simulink model "MCS_STD_FSBB_MODEL_2022b"  (R2022b)
settings: Solver=VariableStepAuto  StartTime=0.0  StopTime=2  RelTol=1e-3
PostLoadFcn:
  | gmp_model_file=get_param(bdroot,'FileName'); if isempty(gmp_model_file), error('GMP:SDPE:ModelPath','The model must be saved before SDPE initialization.'); end; gmp_model_dir=fileparts(gmp_model_file); run(fullfile(gmp_model_dir,'sdpe_mgr','ctrl_settings_matlab_init.m')); gmp_matlab_release=matlabRelease; gmp_repo_root=fullfile(gmp_model_dir,'..','..','..','..','..'); addpath(fullfile(gmp_repo_root,'slib','install_path',gmp_matlab_release.Release,'src')); clear gmp_model_file gmp_model_dir gmp_matlab_release gmp_repo_root;
InitFcn:
  | gmp_model_file=get_param(bdroot,'FileName'); if isempty(gmp_model_file), error('GMP:SDPE:ModelPath','The model must be saved before SDPE initialization.'); end; gmp_model_dir=fileparts(gmp_model_file); run(fullfile(gmp_model_dir,'sdpe_mgr','ctrl_settings_matlab_init.m')); gmp_matlab_release=matlabRelease; gmp_repo_root=fullfile(gmp_model_dir,'..','..','..','..','..'); addpath(fullfile(gmp_repo_root,'slib','install_path',gmp_matlab_release.Release,'src')); clear gmp_model_file gmp_model_dir gmp_matlab_release gmp_repo_root;
undefined symbols (not defined in the file or in its folder): CTRL_ADC_RESOLUTION, CTRL_ADC_VOLTAGE_REF, CTRL_FSBB_IIN_BIAS, CTRL_FSBB_IIN_SENSITIVITY, CTRL_FSBB_IL_BIAS, CTRL_FSBB_IL_SENSITIVITY, CTRL_FSBB_IOUT_BIAS, CTRL_FSBB_IOUT_SENSITIVITY, CTRL_FSBB_VIN_BIAS, CTRL_FSBB_VIN_SENSITIVITY, CTRL_FSBB_VOUT_BIAS, CTRL_FSBB_VOUT_SENSITIVITY, CTRL_PWM_CMP_MAX, CTRL_PWM_DEADBAND_CMP, FSBB_INPUT_VOLTAGE_NOMINAL, FSBB_MODEL_DIODE_RON, FSBB_MODEL_DIODE_VF, FSBB_MODEL_MOSFET_RON, FSBB_MODEL_SNUBBER_C, FSBB_MODEL_SNUBBER_R, FSBB_MODEL_SWITCH_LON, FSBB_PARAM_CIN, FSBB_PARAM_CIN_ESR, FSBB_PARAM_COUT, FSBB_PARAM_COUT_ESR, FSBB_PARAM_L, FSBB_PARAM_L_ESR, FSBB_PARAM_RLOAD_MIN, PWM_FREQ
libraries: gmp_peripheral_utilities x4, spsSeriesRLCBranchLib x4, gmp_std_model_pck x3, spsControlledVoltageSourceLib x1, gmp_sil_core_pack x1, spsGroundLib x1, spspowerguiLib x1
settings Model: SimulationMode=accelerator  Creator=javnson  LastModifiedBy=javnson
settings OptimizationCC: ReuseModelBlockBuffer=on
settings RTWCC: GPUComputeCapability=5.0

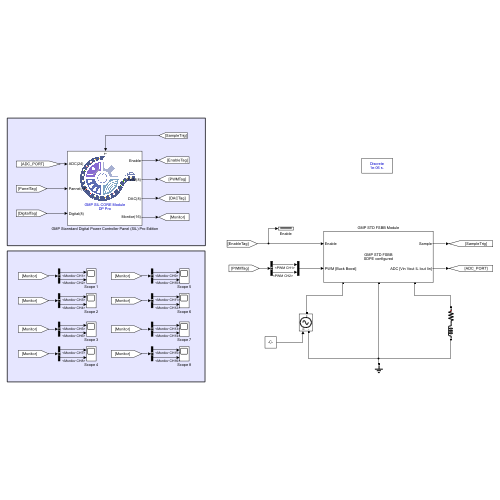
[thumbnail: Simulink's stored preview of the top-level diagram]
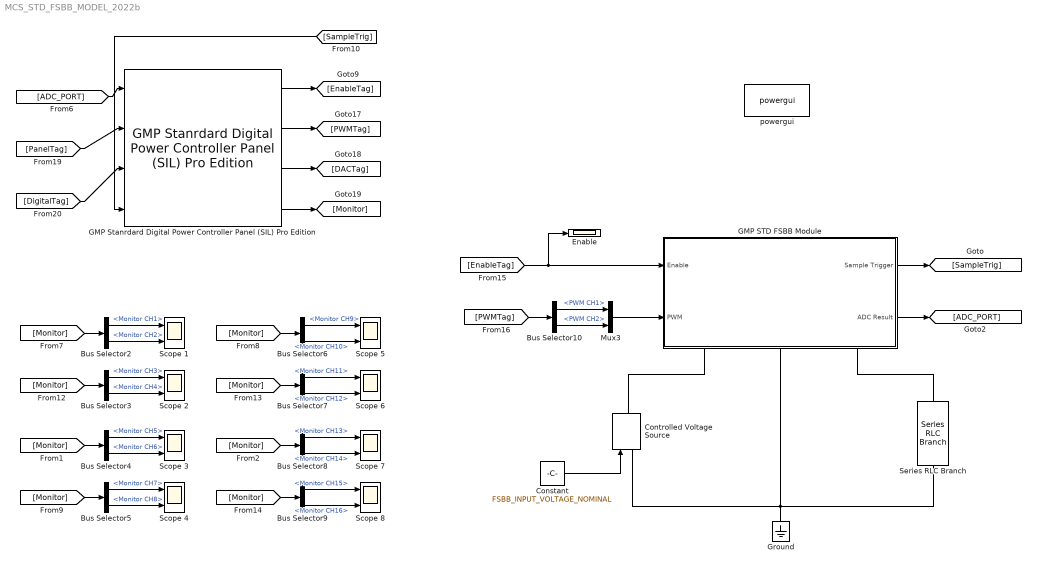
== system MCS_STD_FSBB_MODEL_2022b ==
  Bus Selector10 : BusSelector  OutputSignals=PWM CH1,PWM CH2
  Bus Selector2 : BusSelector  OutputSignals=Monitor CH1,Monitor CH2
  Bus Selector3 : BusSelector  OutputSignals=Monitor CH3,Monitor CH4
  Bus Selector4 : BusSelector  OutputSignals=Monitor CH5,Monitor CH6
  Bus Selector5 : BusSelector  OutputSignals=Monitor CH7,Monitor CH8
  Bus Selector6 : BusSelector  OutputSignals=Monitor CH9,Monitor CH10
  Bus Selector7 : BusSelector  OutputSignals=Monitor CH11,Monitor CH12
  Bus Selector8 : BusSelector  OutputSignals=Monitor CH13,Monitor CH14
  Bus Selector9 : BusSelector  OutputSignals=Monitor CH15,Monitor CH16
  Constant : Constant  Value=FSBB_INPUT_VOLTAGE_NOMINAL
  Controlled Voltage Source : spsControlledVoltageSourceLib/Controlled Voltage Source  Initialize=on  Source_Type=AC  Amplitude=0  Phase=0  Frequency=0  Measurements=None
  Enable : Scope
  GMP STD FSBB Module : Subsystem  mask{Switching_Frequency=PWM_FREQ, PWM_Compare_Max=CTRL_PWM_CMP_MAX, Deadband_Compare=CTRL_PWM_DEADBAND_CMP, Phase_Shift=0, Main_Inductance=FSBB_PARAM_L, Inductor_ESR=FSBB_PARAM_L_ESR, Input_Capacitance=FSBB_PARAM_CIN, Input_Capacitor_ESR=FSBB_PARAM_CIN_ESR, Output_Capacitance=FSBB_PARAM_COUT, Output_Capacitor_ESR=FSBB_PARAM_COUT_ESR, MOSFET_Ron=FSBB_MODEL_MOSFET_RON, Switch_Lon=FSBB_MODEL_SWITCH_LON, Diode_Ron=FSBB_MODEL_DIODE_RON, Diode_Vf=FSBB_MODEL_DIODE_VF, Snubber_R=FSBB_MODEL_SNUBBER_R, Snubber_C=FSBB_MODEL_SNUBBER_C, ADC_Bits=CTRL_ADC_RESOLUTION, ADC_Reference=CTRL_ADC_VOLTAGE_REF, ADC_Initial_Value=0, Vin_Sensor_Gain=CTRL_FSBB_VIN_SENSITIVITY, Vin_Sensor_Bias=CTRL_FSBB_VIN_BIAS, Vout_Sensor_Gain=CTRL_FSBB_VOUT_SENSITIVITY, Vout_Sensor_Bias=CTRL_FSBB_VOUT_BIAS, IL_Sensor_Gain=CTRL_FSBB_IL_SENSITIVITY, IL_Sensor_Bias=CTRL_FSBB_IL_BIAS, Iout_Sensor_Gain=CTRL_FSBB_IOUT_SENSITIVITY, Iout_Sensor_Bias=CTRL_FSBB_IOUT_BIAS, Iin_Sensor_Gain=CTRL_FSBB_IIN_SENSITIVITY, Iin_Sensor_Bias=CTRL_FSBB_IIN_BIAS}
      mask prompts: Switching_Frequency "Switching frequency (Hz)"; PWM_Compare_Max "PWM compare maximum"; Deadband_Compare "Deadband (compare counts)"; Phase_Shift "Phase shift (deg)"; Main_Inductance "Main inductance (H)"; Inductor_ESR "Inductor ESR (Ohm)"; Input_Capacitance "Input capacitance (F)"; Input_Capacitor_ESR "Input capacitor ESR (Ohm)"; Output_Capacitance "Output capacitance (F)"; Output_Capacitor_ESR "Output capacitor ESR (Ohm)"; MOSFET_Ron "MOSFET on resistance (Ohm)"; Switch_Lon "Switch series inductance (H)"; Diode_Ron "Body-diode on resistance (Ohm)"; Diode_Vf "Body-diode forward voltage (V)"; Snubber_R "Snubber resistance (Ohm)"; Snubber_C "Snubber capacitance (F)"; ADC_Bits "ADC resolution (bits)"; ADC_Reference "ADC reference (V)"; ADC_Initial_Value "Sample-and-hold initial value"; Vin_Sensor_Gain "Input-voltage sensitivity (V/V)"; Vin_Sensor_Bias "Input-voltage bias (V)"; Vout_Sensor_Gain "Output-voltage sensitivity (V/V)"; Vout_Sensor_Bias "Output-voltage bias (V)"; IL_Sensor_Gain "Inductor-current sensitivity (V/A)"; IL_Sensor_Bias "Inductor-current bias (V)"; Iout_Sensor_Gain "Boost-side/output-current sensitivity (V/A)"; Iout_Sensor_Bias "Boost-side/output-current bias (V)"; Iin_Sensor_Gain "Buck-side/input-current sensitivity (V/A)"; Iin_Sensor_Bias "Buck-side/input-current bias (V)"
      mask help: SDPE-configured four-switch buck-boost plant. ADC output order: Vin, Vout, IL, Iout (Boost side), Iin (Buck side).
      settings: PortSchema="{\"entries\":[{\"content\":{\"sides\":[{\"content\":{\"connectorIds\":[\"In1\",\"In2\"]},\"type\":\"ConnectorPlacement.EquallySpacedRectSide\",\"uuid\":\"d5d2152c-95da-402f-99b0-c218dbe2e5b0\"},{\"content\":{\"connectorIds\":[\"Out1\",\"Out2\"],\"side\":\"RIGHT\"},\"type\":\"ConnectorPlacement.EquallySpacedRectSide\",\"uuid\":\"d6dcb103-1a45-4ef6-9907-93a1989d933d\"},{\"content\":{\"side\":\"TOP\"},\"type\":\"ConnectorPlacement.EquallySpacedRectSide\",\"uuid\":\"e6268914-9f06-47c0-ace2-6fbd0fa30956\"},{\"content\":{\"connectorIds\":[\"RConn1\",\"RConn2\",\"RConn3\"],\"side\":\"BOTTOM\"},\"type\":\"ConnectorPlacement.EquallySpacedRectSide\",\"uuid\":\"d75aaae5-4ace-4756-8126-8df6a2fa5cb9\"}]},\"type\":\"ConnectorPlacement.EquallySpacedConnector\",\"uuid\":\"07c59de5-034f-4952-94ab-3f04d206adfb\"}],\"packageUris\":[\"http://schema.mathworks.com/mf0/Connector/R2020b\"],\"version\":\"1.0\"}"
      mask DialogControl PWMConfiguration_Group Prompt: PWM Configuration
      mask DialogControl PowerStage_Group Prompt: Power Stage
      mask DialogControl SemiconductorModel_Group Prompt: Semiconductor Model
      mask DialogControl ADCConfiguration_Group Prompt: ADC Configuration
      mask DialogControl VoltageSensors_Group Prompt: Voltage Sensors
      mask DialogControl CurrentSensors_Group Prompt: Current Sensors
      mask Display:
      | disp('GMP STD FSBB\nSDPE configured');
      | port_label('input',1,'Enable'); port_label('input',2,'PWM [Buck Boost]');
      | port_label('output',1,'Sample'); port_label('output',2,'ADC [Vin Vout IL Iout Iin]');
  GMP Stanrdard Digital Power Controller Panel (SIL) Pro Edition : gmp_sil_core_pack/GMP Stanrdard Digital Power Controller Panel (SIL) Pro Edition
      settings: SourceProductName=GMP SIL Core Utilities
  Ground : spsGroundLib/Ground  LConnTagsString=a
  Mux3 : Mux  Inputs=2
  Scope {1..8} (8 alike) : Scope  NumInputPorts=2
  Series RLC Branch : spsSeriesRLCBranchLib/Series RLC Branch  LConnTagsString=__new0  RConnTagsString=__new0  BranchType=RL  Resistance=FSBB_PARAM_RLOAD_MIN  Inductance=10E-6  SetiL0=off  InitialCurrent=0  Capacitance=1e-6  Setx0=off  InitialVoltage=0  Measurements=None
  powergui : spspowerguiLib/powergui  Priority=1  SimulationMode=Discrete  SampleTime=1e-6  frequency=60  Iterations=50  frequencyindice=0  Pbase=100e6  ErrMax=1e-4  UnitsV=kV  UnitsW=MW  buscounter=0  FunctionMessages=off  echomessages=off  EnableUseOfTLC=off  CurrentSourceSwitches=off  DisableSnubberDevices=off  DisableRonSwitches=off  DisableVfSwitches=off  DisplayEquations=off  AutomaticDiscreteSolvers=off  SolverType=Tustin/Backward Euler (TBE)  Interpol=off  ExternalGateDelay=off  methode=off  Ts=100  x0status=blocks  SPID=on  SwTol=0  HookPort=off  NonlinearTolerance=1e-4  nMaxIteration=100  ContinueOnMaxIteration=off  RestoreLinks=warning  ResistiveCurrentMeasurement=off  Frange=[0:2:500]  Ylog=off  Xlog=on  ShowGrid=off  save=off  variable=ZData  structure=0  ZoomFFT=off  StartTime=0.0  cycles=1  DisplayStyle=1  fundamental=60  FreqAxis=off  MaxFrequency=1000  frequencyindicesteady=1  RmsSteady=1  display=off
  wires:
  [PanelTag] -> GMP Stanrdard Digital Power Controller Panel (SIL) Pro Edition/2
  [SampleTrig] -> GMP Stanrdard Digital Power Controller Panel (SIL) Pro Edition/4
  GMP Stanrdard Digital Power Controller Panel (SIL) Pro Edition/2 -> [PWMTag]
  [ADC_PORT] -> GMP Stanrdard Digital Power Controller Panel (SIL) Pro Edition/1
  GMP Stanrdard Digital Power Controller Panel (SIL) Pro Edition/4 -> [Monitor]
  GMP Stanrdard Digital Power Controller Panel (SIL) Pro Edition/1 -> [EnableTag]
  GMP Stanrdard Digital Power Controller Panel (SIL) Pro Edition/3 -> [DACTag]
  [DigitalTag] -> GMP Stanrdard Digital Power Controller Panel (SIL) Pro Edition/3
  Bus Selector8/2 -> Scope 7/2  "<Monitor CH14>"
  Bus Selector2/2 -> Scope 1/2  "<Monitor CH2>"
  Bus Selector4/2 -> Scope 3/2  "<Monitor CH6>"
  Bus Selector3/1 -> Scope 2/1  "<Monitor CH3>"
  [Monitor] -> Bus Selector4/1
  [Monitor] -> Bus Selector7/1
  Bus Selector2/1 -> Scope 1/1  "<Monitor CH1>"
  Bus Selector5/1 -> Scope 4/1  "<Monitor CH7>"
  [Monitor] -> Bus Selector3/1
  Bus Selector8/1 -> Scope 7/1  "<Monitor CH13>"
  Bus Selector3/2 -> Scope 2/2  "<Monitor CH4>"
  Bus Selector4/1 -> Scope 3/1  "<Monitor CH5>"
  Bus Selector7/1 -> Scope 6/1  "<Monitor CH11>"
  [Monitor] -> Bus Selector5/1
  [Monitor] -> Bus Selector8/1
  [Monitor] -> Bus Selector6/1
  Bus Selector6/1 -> Scope 5/1  "<Monitor CH9>"
  Bus Selector5/2 -> Scope 4/2  "<Monitor CH8>"
  [Monitor] -> Bus Selector2/1
  Bus Selector7/2 -> Scope 6/2  "<Monitor CH12>"
  Bus Selector6/2 -> Scope 5/2  "<Monitor CH10>"
  Bus Selector9/1 -> Scope 8/1  "<Monitor CH15>"
  [Monitor] -> Bus Selector9/1
  Bus Selector9/2 -> Scope 8/2  "<Monitor CH16>"
  GMP STD FSBB Module/1(Sample Trigger) -> [SampleTrig]
  GMP STD FSBB Module/2(ADC Result) -> [ADC_PORT]
  [EnableTag] -> GMP STD FSBB Module/1(Enable), Enable/1
  Bus Selector10/1 -> Mux3/1  "<PWM CH1>"
  Bus Selector10/2 -> Mux3/2  "<PWM CH2>"
  Mux3/1 -> GMP STD FSBB Module/2(PWM)
  [PWMTag] -> Bus Selector10/1
  Constant/1 -> Controlled Voltage Source/1
  connections:
  Controlled Voltage Source/RConn1 -- GMP STD FSBB Module/RConn1
  Series RLC Branch/RConn1 -- GMP STD FSBB Module/RConn2 -- Ground/LConn1 -- Controlled Voltage Source/LConn1
  Series RLC Branch/LConn1 -- GMP STD FSBB Module/RConn3

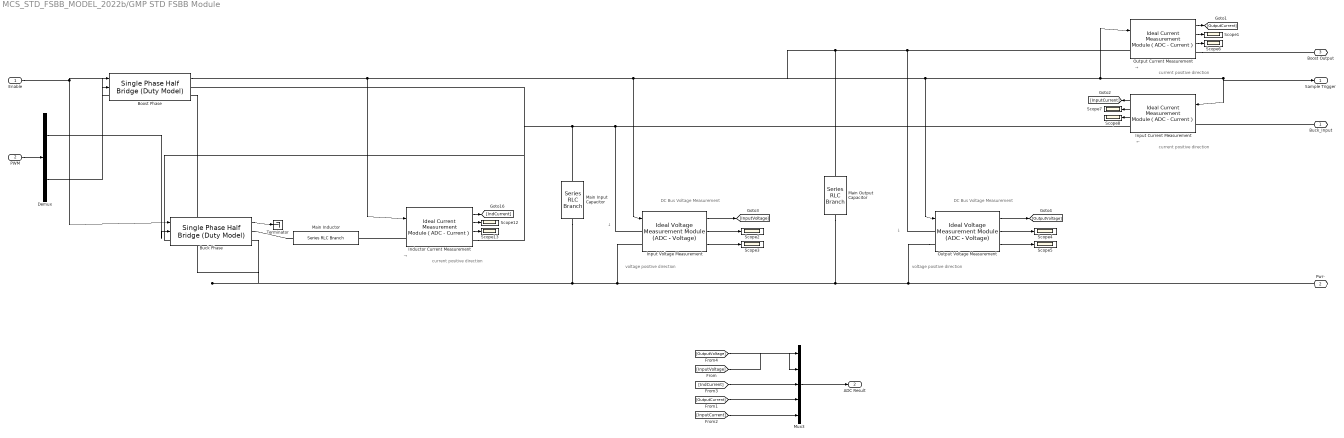
== system MCS_STD_FSBB_MODEL_2022b/GMP STD FSBB Module ==
  note: →
  note: current positive direction
  note: DC Bus Voltage Measurement
  note: ↓
  note: voltage positive direction
  note: voltage positive direction
  note: ↓
  note: DC Bus Voltage Measurement
  note: current positive direction
  note: →
  note: ←
  note: current positive direction
  Enable : Inport
  PWM : Inport  Port=2
  Boost Phase : gmp_peripheral_utilities/Single Phase Half Bridge (Duty Model)  fswitch=Switching_Frequency  CMP_MAX=PWM_Compare_Max  Deadband_Upper=Deadband_Compare  Deadband_Lower=Deadband_Compare  Deadband_us=NaN  phase_shift=Phase_Shift  R_mosfet_on=MOSFET_Ron  Lon=Switch_Lon  Rd=Diode_Ron  Vf=Diode_Vf  Rs=Snubber_R  Cs=Snubber_C
      settings: SourceProductName=Virtual Peripheral Utilities
  Buck Phase : gmp_peripheral_utilities/Single Phase Half Bridge (Duty Model)  fswitch=Switching_Frequency  CMP_MAX=PWM_Compare_Max  Deadband_Upper=Deadband_Compare  Deadband_Lower=Deadband_Compare  Deadband_us=NaN  phase_shift=Phase_Shift  R_mosfet_on=MOSFET_Ron  Lon=Switch_Lon  Rd=Diode_Ron  Vf=Diode_Vf  Rs=Snubber_R  Cs=Snubber_C
      settings: SourceProductName=Virtual Peripheral Utilities
  Demux : Demux  Outputs=2
  Inductor Current Measurement : gmp_std_model_pck/Buck (GMP STD MDL)/Ideal Current Measurement Module（ADC - Current）  ADC_GAIN=IL_Sensor_Gain  ADC_BIT=ADC_Bits  ADC_REFERENCE=ADC_Reference  ADC_BIAS=IL_Sensor_Bias  ADC_INIT=ADC_Initial_Value
      settings: SourceProductName=GMP Control Plant Utilities
  Input Current Measurement : gmp_std_model_pck/Buck (GMP STD MDL)/Ideal Current Measurement Module（ADC - Current）  ADC_GAIN=Iin_Sensor_Gain  ADC_BIT=ADC_Bits  ADC_REFERENCE=ADC_Reference  ADC_BIAS=Iin_Sensor_Bias  ADC_INIT=ADC_Initial_Value
      settings: SourceProductName=GMP Control Plant Utilities
  Input Voltage Measurement : gmp_peripheral_utilities/Ideal Voltage Measurement Module (ADC - Voltage)  ADC_GAIN=Vin_Sensor_Gain  ADC_BIT=ADC_Bits  ADC_REFERENCE=ADC_Reference  ADC_BIAS=Vin_Sensor_Bias  ADC_INIT=ADC_Initial_Value
      settings: SourceProductName=Virtual Peripheral Utilities
  Main Inductor : spsSeriesRLCBranchLib/Series RLC Branch  LConnTagsString=__new0  RConnTagsString=__new0  BranchType=RL  Resistance=Inductor_ESR  Inductance=Main_Inductance  SetiL0=off  InitialCurrent=0  Capacitance=1e-6  Setx0=off  InitialVoltage=0  Measurements=None
  Main Input Capacitor : spsSeriesRLCBranchLib/Series RLC Branch  LConnTagsString=__new0  RConnTagsString=__new0  BranchType=RC  Resistance=Input_Capacitor_ESR  Inductance=1e-3  SetiL0=off  InitialCurrent=0  Capacitance=Input_Capacitance  Setx0=off  InitialVoltage=0  Measurements=None
  Main Output Capacitor : spsSeriesRLCBranchLib/Series RLC Branch  LConnTagsString=__new0  RConnTagsString=__new0  BranchType=RC  Resistance=Output_Capacitor_ESR  Inductance=1e-3  SetiL0=off  InitialCurrent=0  Capacitance=Output_Capacitance  Setx0=off  InitialVoltage=0  Measurements=None
  Mux3 : Mux  Inputs=5
  Output Current Measurement : gmp_std_model_pck/Buck (GMP STD MDL)/Ideal Current Measurement Module（ADC - Current）  ADC_GAIN=Iout_Sensor_Gain  ADC_BIT=ADC_Bits  ADC_REFERENCE=ADC_Reference  ADC_BIAS=Iout_Sensor_Bias  ADC_INIT=ADC_Initial_Value
      settings: SourceProductName=GMP Control Plant Utilities
  Output Voltage Measurement : gmp_peripheral_utilities/Ideal Voltage Measurement Module (ADC - Voltage)  ADC_GAIN=Vout_Sensor_Gain  ADC_BIT=ADC_Bits  ADC_REFERENCE=ADC_Reference  ADC_BIAS=Vout_Sensor_Bias  ADC_INIT=ADC_Initial_Value
      settings: SourceProductName=Virtual Peripheral Utilities
  Scope{1..8,12..13} (10 alike) : Scope
  Terminator : Terminator
  Buck_Input : PMIOPort  Side=Right
  Pwr- : PMIOPort  Port=2  Side=Right
  Boost Output : PMIOPort  Port=3  Side=Right
  Sample Trigger : Outport
  ADC Result : Outport  Port=2
  wires:
  Output Current Measurement/1 -> [OutputCurrent]
  Input Voltage Measurement/3 -> Scope3/1
  Inductor Current Measurement/3 -> Scope13/1
  Mux3/1 -> ADC Result/1
  Buck Phase/1 -> Terminator/1
  Input Current Measurement/1 -> [InputCurrent]
  Output Current Measurement/2 -> Scope1/1
  Enable/1 -> Buck Phase/1, Boost Phase/1
  Input Voltage Measurement/2 -> Scope2/1
  Output Voltage Measurement/3 -> Scope5/1
  Boost Phase/1 -> Inductor Current Measurement/1, Input Voltage Measurement/1, Output Voltage Measurement/1, Output Current Measurement/1, Sample Trigger/1, Input Current Measurement/1
  Inductor Current Measurement/1 -> [IndCurrent]
  Input Voltage Measurement/1 -> [InputVoltage]
  Output Voltage Measurement/2 -> Scope4/1
  PWM/1 -> Demux/1
  Inductor Current Measurement/2 -> Scope12/1
  Input Current Measurement/2 -> Scope7/1
  Input Current Measurement/3 -> Scope8/1
  Output Voltage Measurement/1 -> [OutputVoltage]
  Output Current Measurement/3 -> Scope6/1
  [InputVoltage] -> Mux3/1
  [OutputVoltage] -> Mux3/2
  [IndCurrent] -> Mux3/3
  [OutputCurrent] -> Mux3/4
  [InputCurrent] -> Mux3/5
  Demux/1 -> Buck Phase/2
  Demux/2 -> Boost Phase/2
  connections:
  Main Input Capacitor/LConn1 -- Buck Phase/LConn1 -- Input Current Measurement/RConn1 -- Input Voltage Measurement/LConn1
  Output Voltage Measurement/LConn2 -- Main Output Capacitor/RConn1 -- Input Voltage Measurement/LConn2 -- Main Input Capacitor/RConn1 -- Buck Phase/RConn2 -- Boost Phase/RConn2 -- Pwr-/RConn1
  Inductor Current Measurement/RConn1 -- Boost Phase/RConn1
  Output Voltage Measurement/LConn1 -- Main Output Capacitor/LConn1 -- Boost Phase/LConn1 -- Output Current Measurement/LConn1
  Output Current Measurement/RConn1 -- Boost Output/RConn1
  Main Inductor/RConn1 -- Buck Phase/RConn1
  Buck_Input/RConn1 -- Input Current Measurement/LConn1
  Inductor Current Measurement/LConn1 -- Main Inductor/LConn1
